simulink model "Simulink_DUFF_KK_polynomial"  (R2022a)
settings: Solver=FixedStepAuto  StartTime=0.0  StopTime=Tf  FixedStep=Ts/10  RelTol=1e-3
values from neighbouring files (symbols this model uses):
  A = A(1:n_x,:)    [Duffing_MPC_Evaluation.m]
  B = B(1:n_x,:)    [Duffing_MPC_Evaluation.m]
  eta = 0.001    [Duffing_MPC.m]    (also in Duffing_MPC_Evaluation.m)
  nlobj = nlmpc(nx,ny,nu)    [Duffing_MPC.m]
  ss_0 = Spline_Radial_Obs(x_0,X0)    [Duffing_MPC_Evaluation.m]
  Ts = 1e-2    (= 0.01)    [Duffing_MPC.m]    (also in duff_osc_gen.m)
undefined symbols (not defined in the file or in its folder): C, D
libraries: simulink x1
settings Model: Creator=sergiovaneg  LastModifiedBy=sergiovaneg

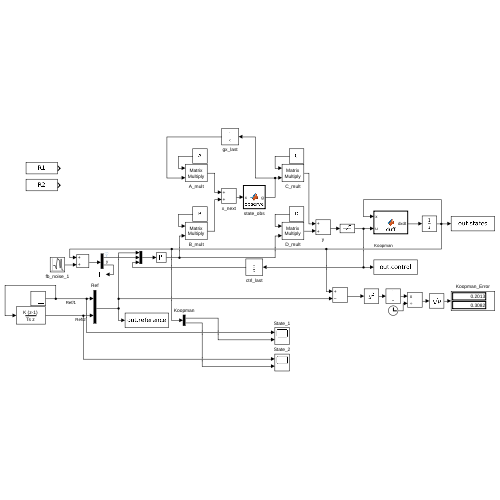
[thumbnail: Simulink's stored preview of the top-level diagram]
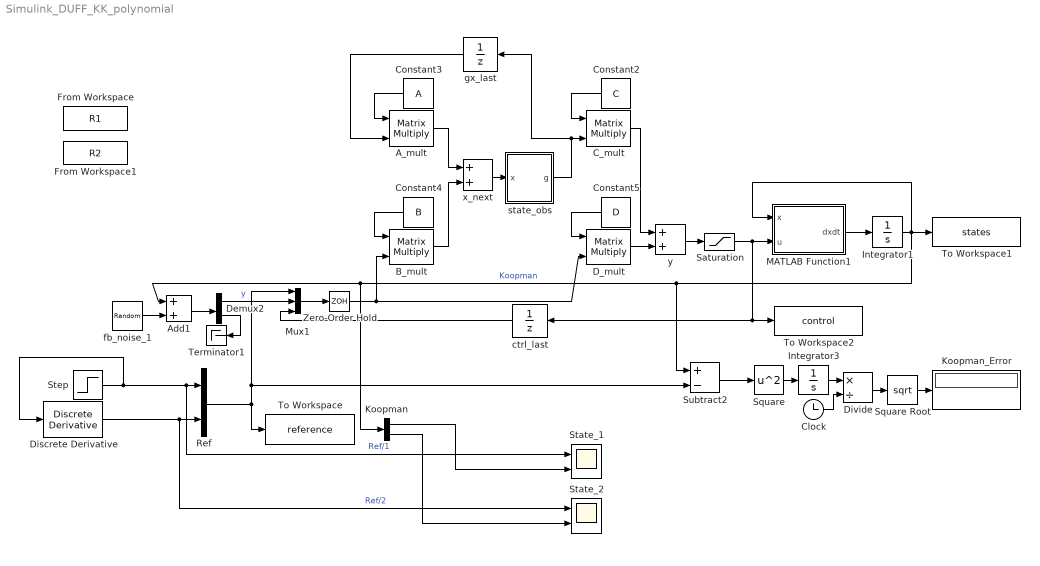
== system Simulink_DUFF_KK_polynomial ==
  A_mult : Product  Multiplication=Matrix(*)
  Add1 : Sum
  B_mult : Product  Multiplication=Matrix(*)
  C_mult : Product  Multiplication=Matrix(*)
  Clock : Clock
  Constant2 : Constant  Value=C  VectorParams1D=off
  Constant3 : Constant  Value=A  VectorParams1D=off
  Constant4 : Constant  Value=B  VectorParams1D=off
  Constant5 : Constant  Value=D  VectorParams1D=off
  D_mult : Product  Multiplication=Matrix(*)
  Demux2 : Demux  Outputs=2
  Discrete Derivative : simulink/Discrete/Discrete Derivative  gainval=1  ICPrevScaledInput=0.0  OutMin=[]  OutMax=[]  OutDataType=fixdt(1, 16)  OutScaling=2^-10  DoSatur=off
  Divide : Product  Inputs=*/
  From Workspace : FromWorkspace  VariableName=R1
  From Workspace1 : FromWorkspace  VariableName=R2
  Integrator1 : Integrator  InitialCondition=zeros(2,1)  UpperSaturationLimit=10  LowerSaturationLimit=-10
  Integrator3 : Integrator
  Koopman : Demux  Outputs=2
  Koopman_Error : Display
      settings: Decimation=3
  MATLAB Function1 : MATLAB Function  TreatAsAtomicUnit=on
  Mux1 : Mux  Inputs=3
  Ref : Mux  Inputs=2
  Saturation : Saturate  UpperLimit=nlobj.MV.Max  LowerLimit=nlobj.MV.Min
  Square : Math  Operator=square
  Square Root : Sqrt
  State_1 : Scope  NumInputPorts=2
  State_2 : Scope  NumInputPorts=2
  Step : Step  Time=0  After=-1  SampleTime=0
  Subtract2 : Sum  Inputs=+-
  Terminator1 : Terminator
  To Workspace : ToWorkspace  VariableName=reference  SampleTime=Ts
      settings: Save2DSignal=2-D array (concatenate along first dimension)
  To Workspace1 : ToWorkspace  VariableName=states  SampleTime=Ts
      settings: Save2DSignal=2-D array (concatenate along first dimension)
  To Workspace2 : ToWorkspace  VariableName=control  SampleTime=Ts
      settings: Save2DSignal=2-D array (concatenate along first dimension)
  Zero-Order Hold : ZeroOrderHold  SampleTime=Ts
  ctrl_last : UnitDelay  SampleTime=Ts  HasFrameUpgradeWarning=on
  fb_noise_1 : RandomNumber  Variance=eta  Seed=[2;3]  SampleTime=Ts
  gx_last : UnitDelay  InitialCondition=ss_0  SampleTime=Ts  HasFrameUpgradeWarning=on
  state_obs : MATLAB Function  TreatAsAtomicUnit=on
  x_next : Sum
  y : Sum
  wires:
  Ref/1 -> Subtract2/2, Mux1/1, To Workspace/1
  Integrator1/1 -> To Workspace1/1, MATLAB Function1/1(x), Subtract2/1, Koopman/1, Add1/1  "Koopman"
  Discrete Derivative/1 -> Ref/2, State_2/1  "Ref/2"
  Saturation/1 -> MATLAB Function1/2(u), ctrl_last/1, To Workspace2/1
  state_obs/1(g) -> gx_last/1, C_mult/2
  Constant4/1 -> B_mult/1
  Constant3/1 -> A_mult/1
  Zero-Order Hold/1 -> D_mult/2, B_mult/2
  x_next/1 -> state_obs/1(x)
  Constant2/1 -> C_mult/1
  Demux2/2 -> Terminator1/1
  C_mult/1 -> y/1
  gx_last/1 -> A_mult/2
  Square/1 -> Integrator3/1
  fb_noise_1/1 -> Add1/2
  ctrl_last/1 -> Mux1/3
  y/1 -> Saturation/1
  Mux1/1 -> Zero-Order Hold/1
  Constant5/1 -> D_mult/1
  MATLAB Function1/1(dxdt) -> Integrator1/1
  Demux2/1 -> Mux1/2  "y"
  D_mult/1 -> y/2
  Add1/1 -> Demux2/1
  A_mult/1 -> x_next/1
  B_mult/1 -> x_next/2
  Subtract2/1 -> Square/1
  Koopman/1 -> State_1/2
  Koopman/2 -> State_2/2
  Square Root/1 -> Koopman_Error/1
  Integrator3/1 -> Divide/1
  Divide/1 -> Square Root/1
  Clock/1 -> Divide/2
  Step/1 -> Discrete Derivative/1, State_1/1, Ref/1  "Ref/1"

== matlab function Simulink_DUFF_KK_polynomial/state_obs ==
  data: x input; g output; expts parameter
function g = observe(x,expts)
    g = ones(size(expts,1),1);
    for i=1:size(g,1)
        for j=1:size(x,1)
            g(i,:) = g(i)*(x(j)^expts(i,j));
        end
    end

== matlab function Simulink_DUFF_KK_polynomial/MATLAB Function1 ==
  data: x input; u input; dxdt output
function dxdt = duff(x,u)
    dxdt = zeros(2,1);
    dxdt(1) = x(2);
    dxdt(2) = x(1)-x(1)^3-0.5*x(2)+u;
